simulink model "Tutorial"  (R2019b)
settings: Solver=VariableStepAuto  StartTime=0.0  StopTime=10.0  RelTol=1e-3
settings Model: Creator=krist  LastModifiedBy=krist

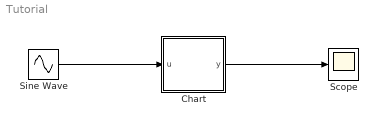
== system Tutorial ==
  Chart : Stateflow chart  BlockKeywords=__PRM__SERIALIZED__DATA__:Stateflow Chart,Stateflow Diagram  TreatAsAtomicUnit=on
  Scope : Scope
  Sine Wave : Sin  SampleTime=0
  wires:
  Sine Wave/1 -> Chart/1(u)
  Chart/1(y) -> Scope/1

== stateflow chart Tutorial/Chart ==
  state ON
    entry: y=1;
  state OFF
    entry: y=-1;
  (default) -> ON
  ON -> OFF : [u<0]
  OFF -> ON : [u>0]
  data: u input; y output
